simulink model "gesamtkonzept_robuster_regler_polbvg"  (R2016b)
settings: Solver=ode1  StartTime=0.0  StopTime=Inf  FixedStep=0.001  RelTol=1e-3
PostLoadFcn:
  | , if any(exist('dsrtsu_mdlpostloadfcn', 'file') == [2, 3, 6]), try dsrtsu_mdlpostloadfcn('Execute', bdroot); catch fprintf('Error in PostLoadFcn (dsrtsu_mdlpostloadfcn) for model "%s":\n %s\n', bdroot, lasterr); end, end,
undefined symbols (not defined in the file): A_b_angle, A_D, B_b_angle, B_D, C_b_angle, C_D, Continuous, D_b_angle, D_D, matA_g, matA_hub_g, matB, matB_g, matB_hub, matB_hub_g, matC_g, matC_hub_g, matE, matE_hub, matR_ges, matR_hub, reglerhub, system, Time
libraries: rti1202lib_dac_class1 x3, rti1202lib_adc_class1 x3, ctrlSharedLib x2, simulink x1, simulink_extras x1, rtiemclib x1, rti1202lib_base x1
(part 2 of 2)

== system gesamtkonzept_robuster_regler_polbvg/RTI Data ==
  RTI Data Store : Subsystem  Tag="struct('private',struct('version',struct('dsVer',uint32(2),'dsVerCreation',uint32(2),'RTI',struct('ver','7.7','type','RTI1202')),'access',struct('type','Model','isPerm',1,'created',['24-Nov-2020 10:16:32'],'modified',['09-Feb-2021 16:18:32'],'location','')),'public',struct('main',struct('data',[]),'sub',struct('name',{{'test_regler_polbvg_aktoren_sensoren_ansprechen'}},'data',{{struct('TH',struct('thTaskInfo',struct('taskType',{'TIMER','HWINT','TMRINT','SWINT','GLINT'},'tasksNumOf',{1,0,0,0,0},'srcIds',{{'TIMERA'},{},{},{},{}},'taskNames',{{['Timer Task 1']},{},{},{},{}})),'th_tc',struct('dataType','TASK','taskGroupId','','taskGroupList',{{}},'taskSchedulingPolicy','FCFS','taskType','TIMER','blkh',-1,'srcId','TIMERA','srcSgnName',['Timer A interrupt'],'srcCpuName','','taskName',['Timer Task 1  [0.001] s'],'taskNameDisplayExt','','smplTime',0.001,'smplTimeOffs',0,'hasFixedPriority',0,'priority',1,'hasFixedOvc',0,'ovcType',1,'ovcMax',1),'tc_th',struct('dataType','TASK','taskGroupId','','taskGroupList',{{}},'taskSchedulingPolicy','FCFS','taskType','TIMER','blkh',-1,'srcId','TIMERA','srcSgnName',['Timer A interrupt'],'srcCpuName','','taskName',['Timer Task 1  [0.001] s'],'taskNameDisplayExt','','smplTime',0.001,'smplTimeOffs',0,'hasFixedPriority',0,'priority',1,'hasFixedOvc',0,'ovcType',1,'ovcMax',1))}})))"  mask(RTI_DATA_STORE){}
      mask help:
      | RTI Data Store Block. This block is used by RTI to store internal model dependent data. Deleting this block will result in data loss.
      |
      | NEVER DELETE, COPY, OR MODIFY THIS BLOCK!
      mask Help:
      | RTI Data Store Block. This block is used by RTI to store internal model dependent data. Deleting this block will result in data loss.
      | 
      | NEVER DELETE, COPY, OR MODIFY THIS BLOCK!
      mask Display: text(0.5, 0.5, ' ', 'HorizontalAlignment', 'center');

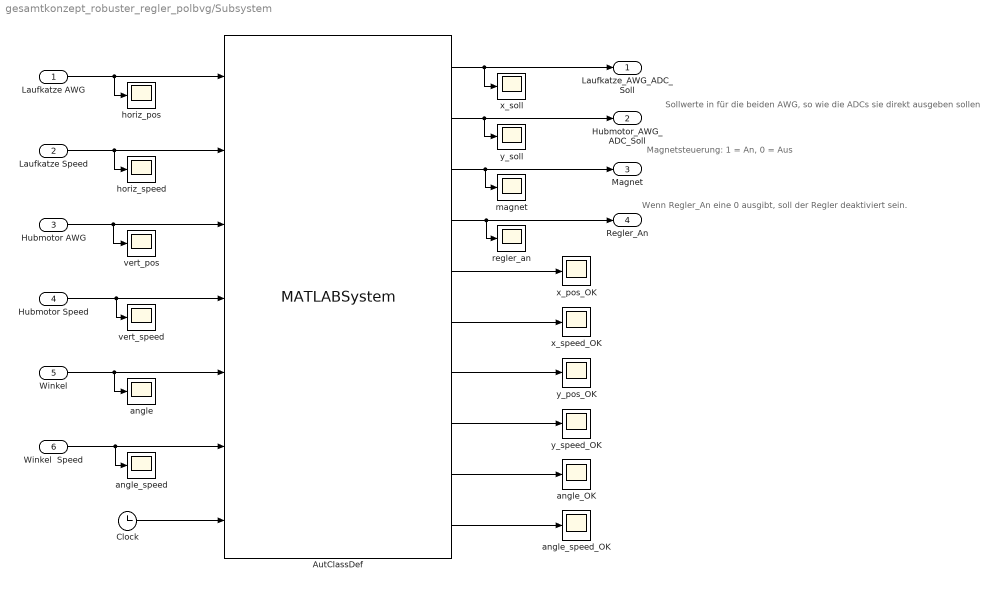
== system gesamtkonzept_robuster_regler_polbvg/Subsystem ==
  note: Magnetsteuerung: 1 = An, 0 = Aus
  note: Sollwerte in für die beiden AWG, so wie die ADCs sie direkt ausgeben sollen
  note: Wenn Regler_An eine 0 ausgibt, soll der Regler deaktiviert sein.
  Laufkatze AWG : Inport  OutMin=0  OutMax=1  OutDataTypeStr=double  PortDimensions=1
  Laufkatze Speed : Inport  Port=2  OutDataTypeStr=double
  Hubmotor AWG : Inport  Port=3  OutMin=0  OutMax=1  OutDataTypeStr=double  PortDimensions=1
  Hubmotor Speed : Inport  Port=4  OutDataTypeStr=double
  Winkel : Inport  Port=5  OutMin=0  OutMax=360  OutDataTypeStr=double  PortDimensions=1
  Winkel  Speed : Inport  Port=6  OutDataTypeStr=double
  AutClassDef : MATLABSystem  System=Steuerung_Automatisierung  start_time=30  add_midpoints=true  midpoint_height=-1  param=param  SimulateUsing=Code generation
      mask Type: Steuerung_Automatisierung
      mask Display:
      | disp('Steuerung_Automatisierung');
      | port_label('input',1,'horiz_pos');
      | port_label('input',2,'horiz_speed');
      | port_label('input',3,'vert_pos');
      | port_label('input',4,'vert_speed');
      | port_label('input',5,'angle');
      | port_label('input',6,'angle_speed');
      | port_label('input',7,'Clock');
      | port_label('output',1,'horiz_setpoint');
      | port_label('output',2,'vert_setpoint');
      | port_label('output',3,'magnet_on');
      | port_label('output',4,'control_enable');
      | port_label('output',5,'x_under_thres');
      | port_label('output',6,'x_speed_under_thres');
      | port_label('output',7,'y_under_thres');
      | port_label('output',8,'y_speed_under_thres');
      | port_label('output',9,'angle_under_thres');
      | port_label('output',10,'angle_speed_under_thres');
  Clock : Clock
  angle : Scope
  angle_OK : Scope
  angle_speed : Scope
  angle_speed_OK : Scope
  horiz_pos : Scope
  horiz_speed : Scope
  magnet : Scope
  regler_an : Scope
  vert_pos : Scope
  vert_speed : Scope
  x_pos_OK : Scope
  x_soll : Scope
  x_speed_OK : Scope
  y_pos_OK : Scope
  y_soll : Scope
  y_speed_OK : Scope
  Laufkatze_AWG_ADC_Soll : Outport
  Hubmotor_AWG_ADC_Soll : Outport  Port=2
  Magnet : Outport  Port=3
  Regler_An : Outport  Port=4
  wires:
  Laufkatze AWG/1 -> AutClassDef/1, horiz_pos/1
  Hubmotor AWG/1 -> AutClassDef/3, vert_pos/1
  Winkel/1 -> AutClassDef/5, angle/1
  AutClassDef/4 -> regler_an/1, Regler_An/1
  AutClassDef/1 -> x_soll/1, Laufkatze_AWG_ADC_Soll/1
  AutClassDef/3 -> Magnet/1, magnet/1
  Clock/1 -> AutClassDef/7
  AutClassDef/2 -> y_soll/1, Hubmotor_AWG_ADC_Soll/1
  AutClassDef/5 -> x_pos_OK/1
  AutClassDef/6 -> x_speed_OK/1
  AutClassDef/7 -> y_pos_OK/1
  AutClassDef/8 -> y_speed_OK/1
  AutClassDef/9 -> angle_OK/1
  AutClassDef/10 -> angle_speed_OK/1
  Laufkatze Speed/1 -> AutClassDef/2, horiz_speed/1
  Hubmotor Speed/1 -> AutClassDef/4, vert_speed/1
  Winkel  Speed/1 -> AutClassDef/6, angle_speed/1

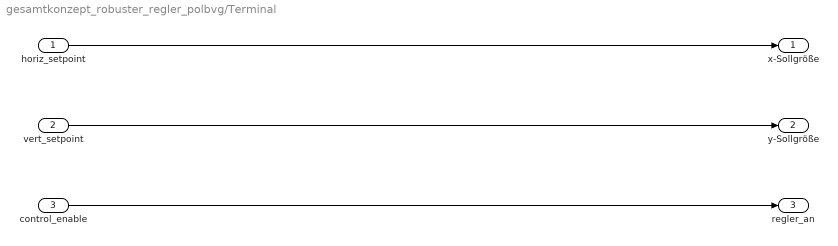
== system gesamtkonzept_robuster_regler_polbvg/Terminal ==
  horiz_setpoint : Inport
  vert_setpoint : Inport  Port=2
  control_enable : Inport  Port=3
  x-Sollgröße : Outport
  y-Sollgröße : Outport  Port=2
  regler_an : Outport  Port=3
  wires:
  horiz_setpoint/1 -> x-Sollgröße/1
  vert_setpoint/1 -> y-Sollgröße/1
  control_enable/1 -> regler_an/1

== system gesamtkonzept_robuster_regler_polbvg/kalman_on ==
  In : Inport
  Enable : EnablePort
  Out : Outport
  wires:
  In/1 -> Out/1

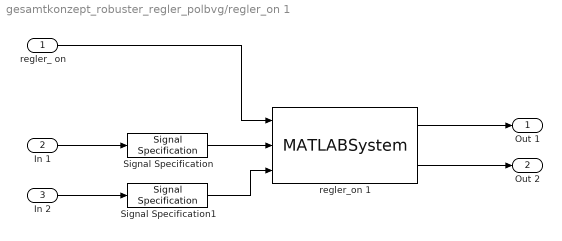
== system gesamtkonzept_robuster_regler_polbvg/regler_on 1 ==
  regler_ on : Inport
  In 1 : Inport  Port=2
  In 2 : Inport  Port=3
  Signal Specification : SignalSpecification  Dimensions=1
  Signal Specification1 : SignalSpecification  Dimensions=1
  regler_on 1 : MATLABSystem  System=regler_switch_2  SimulateUsing=Code generation
      mask Type: regler_switch_2
      mask Display:
      | disp('regler_switch_2');
      | port_label('input',1,'regler_on');
      | port_label('input',2,'input1');
      | port_label('input',3,'input2');
      | port_label('output',1,'y1');
      | port_label('output',2,'y2');
  Out 1 : Outport
  Out 2 : Outport  Port=2
  wires:
  regler_on 1/1 -> Out 1/1
  regler_on 1/2 -> Out 2/1
  In 2/1 -> Signal Specification1/1
  In 1/1 -> Signal Specification/1
  Signal Specification/1 -> regler_on 1/2
  Signal Specification1/1 -> regler_on 1/3
  regler_ on/1 -> regler_on 1/1

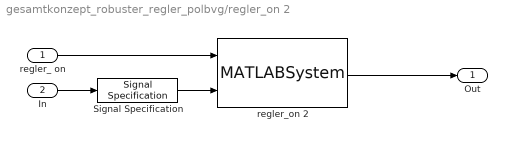
== system gesamtkonzept_robuster_regler_polbvg/regler_on 2 ==
  regler_ on : Inport
  In : Inport  Port=2
  Signal Specification : SignalSpecification  Dimensions=1
  regler_on 2 : MATLABSystem  System=regler_switch_1  SimulateUsing=Code generation
      mask Type: regler_switch_1
      mask Display:
      | disp('regler_switch_1');
      | port_label('input',1,'regler_on');
      | port_label('input',2,'input');
      | port_label('output',1,'y');
  Out : Outport
  wires:
  regler_ on/1 -> regler_on 2/1
  regler_on 2/1 -> Out/1
  Signal Specification/1 -> regler_on 2/2
  In/1 -> Signal Specification/1

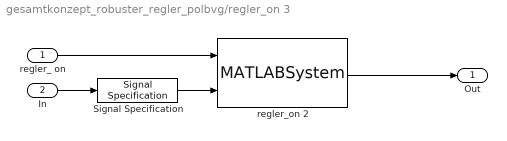
== system gesamtkonzept_robuster_regler_polbvg/regler_on 3 ==
  regler_ on : Inport
  In : Inport  Port=2
  Signal Specification : SignalSpecification  Dimensions=1
  regler_on 2 : MATLABSystem  System=regler_switch_1  SimulateUsing=Code generation
      mask Type: regler_switch_1
      mask Display:
      | disp('regler_switch_1');
      | port_label('input',1,'regler_on');
      | port_label('input',2,'input');
      | port_label('output',1,'y');
  Out : Outport
  wires:
  regler_ on/1 -> regler_on 2/1
  regler_on 2/1 -> Out/1
  Signal Specification/1 -> regler_on 2/2
  In/1 -> Signal Specification/1

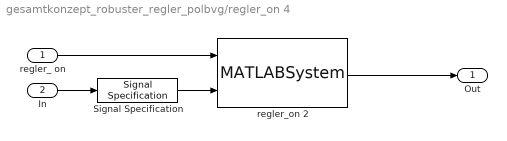
== system gesamtkonzept_robuster_regler_polbvg/regler_on 4 ==
  regler_ on : Inport
  In : Inport  Port=2
  Signal Specification : SignalSpecification  Dimensions=1
  regler_on 2 : MATLABSystem  System=regler_switch_1  SimulateUsing=Code generation
      mask Type: regler_switch_1
      mask Display:
      | disp('regler_switch_1');
      | port_label('input',1,'regler_on');
      | port_label('input',2,'input');
      | port_label('output',1,'y');
  Out : Outport
  wires:
  regler_ on/1 -> regler_on 2/1
  regler_on 2/1 -> Out/1
  Signal Specification/1 -> regler_on 2/2
  In/1 -> Signal Specification/1

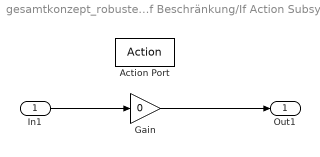
== system gesamtkonzept_robuster_regler_polbvg/Anti-Schlupf Beschränkung/If Action Subsystem ==
  In1 : Inport
  Action Port : ActionPort  ActionType=then
  Gain : Gain  Gain=0
  Out1 : Outport
  wires:
  In1/1 -> Gain/1
  Gain/1 -> Out1/1

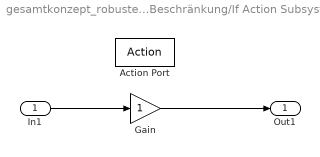
== system gesamtkonzept_robuster_regler_polbvg/Anti-Schlupf Beschränkung/If Action Subsystem1 ==
  In1 : Inport
  Action Port : ActionPort  ActionType=else
  Gain : Gain
  Out1 : Outport
  wires:
  In1/1 -> Gain/1
  Gain/1 -> Out1/1

== system gesamtkonzept_robuster_regler_polbvg/Kalman Filter/Initial State ==
  In : Inport
  Trigger : TriggerPort  VariantControl=Variant
  Out : Outport
  wires:
  In/1 -> Out/1

== system gesamtkonzept_robuster_regler_polbvg/Kalman Filter/kalman_on ==
  In : Inport
  Enable : EnablePort
  Out : Outport
  wires:
  In/1 -> Out/1

== system gesamtkonzept_robuster_regler_polbvg/RTI Data/RTI Data Store ==
  RTI Data Store : Subsystem  mask(RTI_DATA_STORE){}
      mask help:
      | RTI Data Store Block. This block is used by RTI to store internal model dependent data. Deleting this block will result in data loss.
      |
      | NEVER DELETE, COPY, OR MODIFY THIS BLOCK!
      mask Help:
      | RTI Data Store Block. This block is used by RTI to store internal model dependent data. Deleting this block will result in data loss.
      | 
      | NEVER DELETE, COPY, OR MODIFY THIS BLOCK!
      mask Display: text(0.5, 0.5, ' ', 'HorizontalAlignment', 'center');

== system gesamtkonzept_robuster_regler_polbvg/RTI Data/RTI Data Store/RTI Data Store ==
  RTI Data Store : Subsystem  mask(RTI_DATA_STORE){}
      mask help:
      | RTI Data Store Block. This block is used by RTI to store internal model dependent data. Deleting this block will result in data loss.
      |
      | NEVER DELETE, COPY, OR MODIFY THIS BLOCK!
      mask Help:
      | RTI Data Store Block. This block is used by RTI to store internal model dependent data. Deleting this block will result in data loss.
      | 
      | NEVER DELETE, COPY, OR MODIFY THIS BLOCK!
      mask Display: text(0.5, 0.5, ' ', 'HorizontalAlignment', 'center');

== system gesamtkonzept_robuster_regler_polbvg/RTI Data/RTI Data Store/RTI Data Store/RTI Data Store ==
  RTI Data Store : Subsystem  mask(RTI_DATA_STORE){}
      mask help:
      | RTI Data Store Block. This block is used by RTI to store internal model dependent data. Deleting this block will result in data loss.
      |
      | NEVER DELETE, COPY, OR MODIFY THIS BLOCK!
      mask Help:
      | RTI Data Store Block. This block is used by RTI to store internal model dependent data. Deleting this block will result in data loss.
      | 
      | NEVER DELETE, COPY, OR MODIFY THIS BLOCK!
      mask Display: text(0.5, 0.5, ' ', 'HorizontalAlignment', 'center');

== system gesamtkonzept_robuster_regler_polbvg/RTI Data/RTI Data Store/RTI Data Store/RTI Data Store/RTI Data Store ==

== matlab function gesamtkonzept_robuster_regler_polbvg/Umrechnung Sensor ==
  data: theta_sensor input; theta output
function theta  = sensorWinkel(theta_sensor)
% berechnet aus dem gemessenen Winkel den tatsächlichen Winkel des
% Lasthebers

% l_verb: Länge des Verbindungsstücks
% l_welle: Abstand der beiden Wellen

% Parameter für die Winkelumrechnung
l_verb = 0.109; % m %
l_welle = 0.0575; % m %

theta = asin(sin(theta_sensor) * (l_verb / sqrt(l_welle^2 + l_verb^2 - (2 * l_verb * l_welle * cos(theta_sensor)))));

== matlab function gesamtkonzept_robuster_regler_polbvg/Kalman Filter/Berechnung Systemmatrizen ==
  data: matA_ges output; L input; matB_ges output; matC_ges output; matD_ges output; T_K input; K_K input; R input; ue input; g input
function [matA_ges, matB_ges, matC_ges, matD_ges]  = calcSysMatrixStoerGes(L, T_K, K_K, R, ue, g)

% System ohne Störgrößen
matA = [0 1                           0                   0;
        0 -(T_K^-1)            0                   0;
        0 0                           0                   1;
        0 (T_K*L)^-1    -g*(L^-1)   0];

matB = [0; (2*pi*R*K_K)/(ue*T_K); 0; (-2*pi*R*K_K)/(ue*T_K*L)];

matC = [1 0 0 0; 0 0 1 0];


% Störung: Spannungsoffset
% Einfluss der Störung auf Zustände
matE = matB;

% Störmodell
matA_s = 0; % stückweise konstant
matC_s = 1;

% Modell mit Störung 1
matA_g_1 = [matA                      matE*matC_s;
            zeros(1,size(matA,2))     matA_s];

matB_g_1 = [matB; zeros(1,size(matB,2))];

matC_g_1 = [matC zeros(size(matC,1),1)];


% Störung: Winkeloffset
% Einfluss der Störung auf Zustände
matE = [0; 0; 0; 0; 0]; % kein Einfluss auf Zustände, da Winkeloffset erst am Ausgang wirkt

% Störmodell
matA_s = 0; % stückweise konstant
matC_s = 1;


% Gesamtmodell
matA_ges = [matA_g_1                     matE*matC_s;
            zeros(1,size(matA_g_1,2))    matA_s];

matB_ges = [matB_g_1; zeros(1,size(matB_g_1,2))];

matC_ges = [matC_g_1 [0; 1]]; % nicht wie in bsw. RLM mit Nullen aufgefüllt (s.o.), da Störung erst am Ausgang wirkt

matD_ges = [0; 0];


end
